simulink model "IFACS_Spring2026"  (R2025b)
settings: Solver=ode23t  StartTime=0.0  StopTime=3600*24*3  FixedStep=1  RelTol=1e-3  AbsTol=1e-3
values from neighbouring files (symbols this model uses):
  ac_cooling_capacity = 5000    [IFACS_Constants.m]
  ac_power = ac_cooling_capacity / ac_COP    (= 1250)    [IFACS_Constants.m]
  house_H = 6    [IFACS_Constants.m]
  house_L = 20    [IFACS_Constants.m]
  house_W = 10    [IFACS_Constants.m]
  roof_pitch = 15    [IFACS_Constants.m]
  TinIC = 24    [IFACS_Constants.m]
libraries: fl_lib x215, nesl_utility x52, simulink_extras x29, SimscapeFluids_lib x3
(part 5 of 5)

== system IFACS_Spring2026/House Cooled by simple AC unit/House Thermal Network/House Thermal Network/Temp Measurements ==
  Celsius to Fahrenheit : simulink_extras/Transformations/Celsius to Fahrenheit
  Celsius to Fahrenheit1 : simulink_extras/Transformations/Celsius to Fahrenheit
  Celsius to Fahrenheit2 : simulink_extras/Transformations/Celsius to Fahrenheit
  PS2S1 : nesl_utility/PS-Simulink Converter  PhysicalDomain=network_engine_domain  SubClassName=ps_output  LeftPortType=input  RightPortType=output  PseudoPeriodic=off  Frequencies=[]  VectorFormat=1-D array  Unit=degC  AffineConversion=on
  PS2S2 : nesl_utility/PS-Simulink Converter  PhysicalDomain=network_engine_domain  SubClassName=ps_output  LeftPortType=input  RightPortType=output  PseudoPeriodic=off  Frequencies=[]  VectorFormat=1-D array  Unit=degC  AffineConversion=on
  PS2S3 : nesl_utility/PS-Simulink Converter  PhysicalDomain=network_engine_domain  SubClassName=ps_output  LeftPortType=input  RightPortType=output  PseudoPeriodic=off  Frequencies=[]  VectorFormat=1-D array  Unit=degC  AffineConversion=on
  TRef2 : fl_lib/Thermal/Thermal Elements/Thermal Reference
  TRef3 : fl_lib/Thermal/Thermal Elements/Thermal Reference
  TRef4 : fl_lib/Thermal/Thermal Elements/Thermal Reference
  Temperature Sensor1 : fl_lib/Thermal/Thermal Sensors/Temperature Sensor  temperature_measure=foundation.enum.MeasurementReference.difference
  Temperature Sensor2 : fl_lib/Thermal/Thermal Sensors/Temperature Sensor  temperature_measure=foundation.enum.MeasurementReference.difference
  Temperature Sensor3 : fl_lib/Thermal/Thermal Sensors/Temperature Sensor  temperature_measure=foundation.enum.MeasurementReference.difference
  Roof Temp : PMIOPort  Side=Left
  Wall Temp : PMIOPort  Port=2  Side=Left
  Window Temp : PMIOPort  Port=3  Side=Left
  Fahrenheit out : Outport
  Fahrenheit out1 : Outport  Port=2
  Fahrenheit out2 : Outport  Port=3
  wires:
  PS2S3/1 -> Celsius to Fahrenheit2/1  "Window"
  PS2S1/1 -> Celsius to Fahrenheit/1  "Roof"
  PS2S2/1 -> Celsius to Fahrenheit1/1  "Wall"
  Celsius to Fahrenheit2/1 -> Fahrenheit out2/1
  Celsius to Fahrenheit1/1 -> Fahrenheit out1/1
  Celsius to Fahrenheit/1 -> Fahrenheit out/1
  connections:
  PS2S2/LConn1 -- Temperature Sensor2/RConn2
  PS2S3/LConn1 -- Temperature Sensor3/RConn2
  TRef2/LConn1 -- Temperature Sensor1/RConn1
  TRef3/LConn1 -- Temperature Sensor2/RConn1
  PS2S1/LConn1 -- Temperature Sensor1/RConn2
  Temperature Sensor2/LConn1 -- Wall Temp/RConn1
  TRef4/LConn1 -- Temperature Sensor3/RConn1
  Temperature Sensor3/LConn1 -- Window Temp/RConn1
  Temperature Sensor1/LConn1 -- Roof Temp/RConn1

== matlab function IFACS_Spring2026/House Cooled by Singular Fan, Proportional Controller/Fan Parameters/Fan Activation/Inverted Sigmoid Power Function ==
  data: Tmin input; Tenv input; Troom input; Fanpwr output
function Fanpwr = fcn(Tmin, Tenv, Troom)

Fanpwr = -exp(-.5*abs(Troom-Tmin))+1;

if Tmin > Troom || Tenv > Troom
    Fanpwr = 0;
end

== matlab function IFACS_Spring2026/House Cooled by AC and Singular Fan, Proportional Controller/Fan Parameters/Fan Activation/Inverted Sigmoid Power Function ==
  data: Tmin input; Tenv input; Troom input; Fanpwr output
function Fanpwr = fcn(Tmin, Tenv, Troom)

Fanpwr = -exp(-.5*abs(Troom-Tmin))+1;

if Tmin > Troom || Tenv > Troom
    Fanpwr = 0;
end
